simulink model "sample_model_20231101_1"  (R2023b)
settings: Solver=VariableStepAuto  StartTime=0.0  StopTime=10.0  RelTol=1e-3
settings Model: Creator=lisjyw  LastModifiedBy=lisjyw

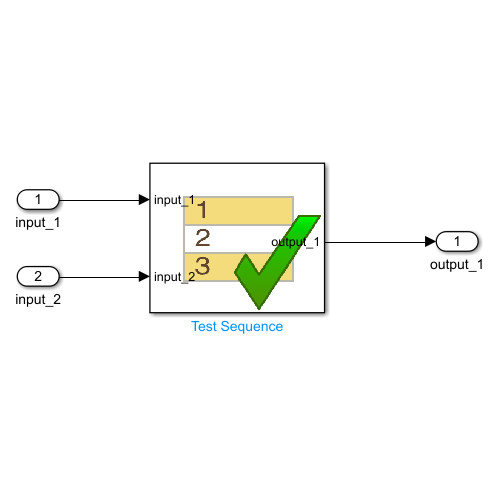
[thumbnail: Simulink's stored preview of the top-level diagram]
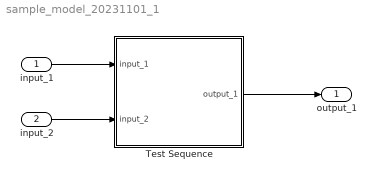
== system sample_model_20231101_1 ==
  input_1 : Inport
  input_2 : Inport  Port=2
  Test Sequence : Test Sequence  TreatAsAtomicUnit=on
  output_1 : Outport
  wires:
  input_1/1 -> Test Sequence/1(input_1)
  input_2/1 -> Test Sequence/2(input_2)
  Test Sequence/1(output_1) -> output_1/1

== stateflow chart sample_model_20231101_1/Test Sequence ==
  state step_1
    output_1 = input_1*input_2;
  (default) -> step_1
  data: input_1 input; input_2 input; output_1 output
